simulink model "ActiveSupensionTS"  (R2014a)
settings: Solver=ode45  StartTime=0.0  StopTime=10.0  RelTol=1e-3
undefined symbols (not defined in the file): A1, A2, I4
libraries: fuzblock x1
settings Model: Creator=MLRida  LastModifiedBy=MLRida

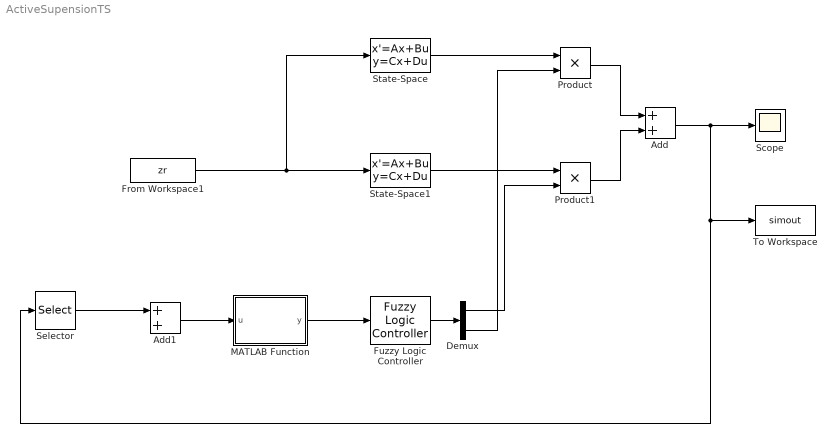
== system ActiveSupensionTS ==
  Add : Sum
  Add1 : Sum
  Demux : Demux  Outputs=2
  From Workspace1 : FromWorkspace  VariableName=zr  SampleTime=0
  Fuzzy Logic Controller : fuzblock/Fuzzy Logic  Controller  fis=TS_model
  MATLAB Function : MATLAB Function  TreatAsAtomicUnit=on
  Product : Product
  Product1 : Product
  Scope : Scope
  Selector : Selector  InputPortWidth=4  Indices=[1 3]
  State-Space : StateSpace  A=A1  B=I4  C=I4  D=0  X0=0
  State-Space1 : StateSpace  A=A2  B=I4  C=I4  D=0  X0=0
  To Workspace : ToWorkspace  VariableName=simout  SaveFormat=Timeseries  SampleTime=-1
  wires:
  From Workspace1/1 -> State-Space/1, State-Space1/1
  State-Space/1 -> Product/1
  State-Space1/1 -> Product1/1
  Demux/1 -> Product1/2
  Demux/2 -> Product/2
  Fuzzy Logic Controller/1 -> Demux/1
  MATLAB Function/1(y) -> Fuzzy Logic Controller/1
  Add1/1 -> MATLAB Function/1(u)
  Product/1 -> Add/1
  Product1/1 -> Add/2
  Add/1 -> Selector/1, To Workspace/1, Scope/1
  Selector/1 -> Add1/1

== matlab function ActiveSupensionTS/MATLAB Function ==
  data: u input; y output
function y = fcn(u)
%#codegen

y = u;
